simulink library "libIntegratorModel"  (R2020b)
settings: Solver=VariableStepAuto  StartTime=0.0  StopTime=10.0  RelTol=1e-3
undefined symbols (not defined in the file): outputs
settings Model: Creator=caatay  LastModifiedBy=caatay

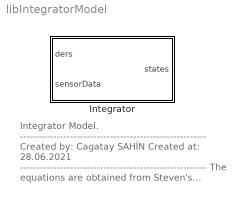
== system libIntegratorModel ==
  note: Integrator Model.
      | --------------------------------------------------------
      | Created by: Cagatay SAHİN
      | Created at: 28.06.2021
      | --------------------------------------------------------
      | The equations are obtained from
      | Steven's textbook.
      | The reference book can be found in
      | "references folder".
      | --------------------------------------------------------
      | for question:
      | cagataysahin44@gmail.com
  Integrator : Subsystem  mask(Flight Control System Module - Integrator){outputs=outputs}
      mask prompts: outputs "Trimmed States"
      mask help: Integrator module is used for integration of state derivatives. Also ther are some sensor information that must be consider as state information. Thus, these values are used in this module.
      mask Help:
      | This block integrate state derivative to state variables.
      | -------------------------------------------------------------------------------------------------------------------------------------------------
      | Inputs of this block set are:
      | 	ders: Derivative Information of states
      | 	sensorData: Sensor data information of states.
      | Outputs of this block set are:
      | 	states: State Information.
      | -------------------------------------------------------------------------------------------------------------------------------------------------
      | For question: "cagataysahin44@gmail.com"
      mask Display:
      | port_label('input',1,'ders','texmode','on');
      | port_label('input',2,'sensorData','texmode','on');
      | 
      | port_label('output',1,'states','texmode','on');

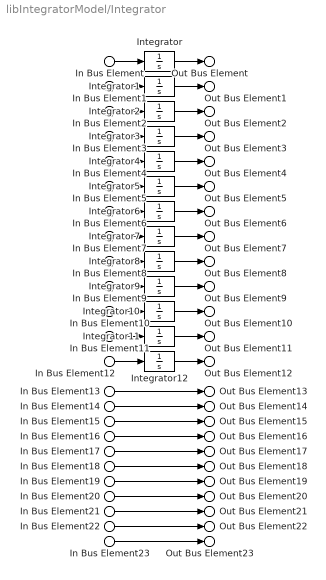
== system libIntegratorModel/Integrator ==
  In Bus Element : Inport  PortName=ders  Element=tas
  In Bus Element1 : Inport  PortName=ders  Element=alpha
  In Bus Element2 : Inport  PortName=ders  Element=beta
  In Bus Element3 : Inport  PortName=ders  Element=phi
  In Bus Element4 : Inport  PortName=ders  Element=theta
  In Bus Element5 : Inport  PortName=ders  Element=psi
  In Bus Element6 : Inport  PortName=ders  Element=p
  In Bus Element7 : Inport  PortName=ders  Element=q
  In Bus Element8 : Inport  PortName=ders  Element=r
  In Bus Element9 : Inport  PortName=ders  Element=x_e
  In Bus Element10 : Inport  PortName=ders  Element=y_e
  In Bus Element11 : Inport  PortName=ders  Element=z_e
  In Bus Element12 : Inport  PortName=ders  Element=power
  In Bus Element13 : Inport  Port=2  PortName=sensorData  Element=u
  In Bus Element14 : Inport  Port=2  PortName=sensorData  Element=v
  In Bus Element15 : Inport  Port=2  PortName=sensorData  Element=w
  In Bus Element16 : Inport  Port=2  PortName=sensorData  Element=q0
  In Bus Element17 : Inport  Port=2  PortName=sensorData  Element=q1
  In Bus Element18 : Inport  Port=2  PortName=sensorData  Element=q2
  In Bus Element19 : Inport  Port=2  PortName=sensorData  Element=q3
  In Bus Element20 : Inport  Port=2  PortName=sensorData  Element=aN
  In Bus Element21 : Inport  Port=2  PortName=sensorData  Element=aY
  In Bus Element22 : Inport  Port=2  PortName=sensorData  Element=lat
  In Bus Element23 : Inport  Port=2  PortName=sensorData  Element=long
  Integrator : Integrator  InitialCondition=outputs.trim.states.tas
  Integrator1 : Integrator  InitialCondition=outputs.trim.states.alpha
  Integrator10 : Integrator  InitialCondition=outputs.trim.states.y_e
  Integrator11 : Integrator  InitialCondition=outputs.trim.states.z_e
  Integrator12 : Integrator  InitialCondition=outputs.trim.states.power
  Integrator2 : Integrator  InitialCondition=outputs.trim.states.beta
  Integrator3 : Integrator  InitialCondition=outputs.trim.states.phi
  Integrator4 : Integrator  InitialCondition=outputs.trim.states.theta
  Integrator5 : Integrator  InitialCondition=outputs.trim.states.psi
  Integrator6 : Integrator  InitialCondition=outputs.trim.states.p
  Integrator7 : Integrator  InitialCondition=outputs.trim.states.q
  Integrator8 : Integrator  InitialCondition=outputs.trim.states.r
  Integrator9 : Integrator  InitialCondition=outputs.trim.states.x_e
  Out Bus Element : Outport  PortName=states  Element=tas
  Out Bus Element1 : Outport  PortName=states  Element=alpha
  Out Bus Element2 : Outport  PortName=states  Element=beta
  Out Bus Element3 : Outport  PortName=states  Element=phi
  Out Bus Element4 : Outport  PortName=states  Element=theta
  Out Bus Element5 : Outport  PortName=states  Element=psi
  Out Bus Element6 : Outport  PortName=states  Element=p
  Out Bus Element7 : Outport  PortName=states  Element=q
  Out Bus Element8 : Outport  PortName=states  Element=r
  Out Bus Element9 : Outport  PortName=states  Element=x_e
  Out Bus Element10 : Outport  PortName=states  Element=y_e
  Out Bus Element11 : Outport  PortName=states  Element=z_e
  Out Bus Element12 : Outport  PortName=states  Element=power
  Out Bus Element13 : Outport  PortName=states  Element=u
  Out Bus Element14 : Outport  PortName=states  Element=v
  Out Bus Element15 : Outport  PortName=states  Element=w
  Out Bus Element16 : Outport  PortName=states  Element=q0
  Out Bus Element17 : Outport  PortName=states  Element=q1
  Out Bus Element18 : Outport  PortName=states  Element=q2
  Out Bus Element19 : Outport  PortName=states  Element=q3
  Out Bus Element20 : Outport  PortName=states  Element=aN
  Out Bus Element21 : Outport  PortName=states  Element=aY
  Out Bus Element22 : Outport  PortName=states  Element=lat
  Out Bus Element23 : Outport  PortName=states  Element=long
  wires:
  In Bus Element/1 -> Integrator/1
  In Bus Element1/1 -> Integrator1/1
  In Bus Element2/1 -> Integrator2/1
  In Bus Element3/1 -> Integrator3/1
  In Bus Element4/1 -> Integrator4/1
  In Bus Element5/1 -> Integrator5/1
  In Bus Element6/1 -> Integrator6/1
  In Bus Element7/1 -> Integrator7/1
  In Bus Element8/1 -> Integrator8/1
  In Bus Element9/1 -> Integrator9/1
  In Bus Element10/1 -> Integrator10/1
  In Bus Element11/1 -> Integrator11/1
  In Bus Element12/1 -> Integrator12/1
  Integrator/1 -> Out Bus Element/1
  Integrator2/1 -> Out Bus Element2/1
  Integrator1/1 -> Out Bus Element1/1
  Integrator3/1 -> Out Bus Element3/1
  Integrator4/1 -> Out Bus Element4/1
  Integrator5/1 -> Out Bus Element5/1
  Integrator6/1 -> Out Bus Element6/1
  Integrator7/1 -> Out Bus Element7/1
  Integrator8/1 -> Out Bus Element8/1
  Integrator9/1 -> Out Bus Element9/1
  Integrator11/1 -> Out Bus Element11/1
  Integrator10/1 -> Out Bus Element10/1
  Integrator12/1 -> Out Bus Element12/1
  In Bus Element13/1 -> Out Bus Element13/1
  In Bus Element14/1 -> Out Bus Element14/1
  In Bus Element15/1 -> Out Bus Element15/1
  In Bus Element16/1 -> Out Bus Element16/1
  In Bus Element17/1 -> Out Bus Element17/1
  In Bus Element18/1 -> Out Bus Element18/1
  In Bus Element19/1 -> Out Bus Element19/1
  In Bus Element20/1 -> Out Bus Element20/1
  In Bus Element21/1 -> Out Bus Element21/1
  In Bus Element22/1 -> Out Bus Element22/1
  In Bus Element23/1 -> Out Bus Element23/1
